simulink model "Assignment2_hardware_hiding"  (R2020a)
settings: Solver=FixedStepAuto  StartTime=0.0  StopTime=inf  FixedStep=1e-3  RelTol=1e-3  EnableMultiTasking=on
undefined symbols (not defined in the file or in its folder): A0, A1, D0, D1, D10, D11, D12, D13, D2, D3, D4, D5, D6, D7, D8, D9, PTA0, PTA1, PTA2, PTB2, PTB23, PTB3, PTB9, PTC16, PTC17, PTC2, PTC3, PTC4, PTD0, PTD1, PTD2, PTD3
libraries: frdmk64flib x22, etargetslib x7
settings Model: ExtModeTrigDuration=5  Creator=iceca  LastModifiedBy=iceca
settings OptimizationCC: EnhancedBackFolding=on  PassReuseOutputArgsAs=Individual arguments  ZeroExternalMemoryAtStartup=off  ZeroInternalMemoryAtStartup=off  MaxStackSize=64  OptimizeBlockOrder=speed  DifferentSizesBufferReuse=on  OptimizationCustomize=off  EfficientTunableParamExpr=on
settings DebuggingCC: ParameterTunabilityLossMsg=error
settings HardwareCC: ProdBitPerPointer=32  ProdBitPerSizeT=32  ProdBitPerPtrDiffT=32  ProdLargestAtomicInteger=Long  ProdLargestAtomicFloat=Double  ProdWordSize=32  ProdHWDeviceType=ARM Compatible->ARM Cortex
settings SFSimCC: MATLABDynamicMemAlloc=off
settings RTWCC: SystemTargetFile=ert.tlc  HardwareBoard=NXP FRDM-K64F  TemplateMakefile=ert_default_tmf  Toolchain=GNU Tools for ARM Embedded Processors
settings CodeAppCC: ForceParamTrailComments=on  IgnoreCustomStorageClasses=off  OperatorAnnotations=on  SimulinkDataObjDesc=on  SFDataObjDesc=on  InsertBlockDesc=on

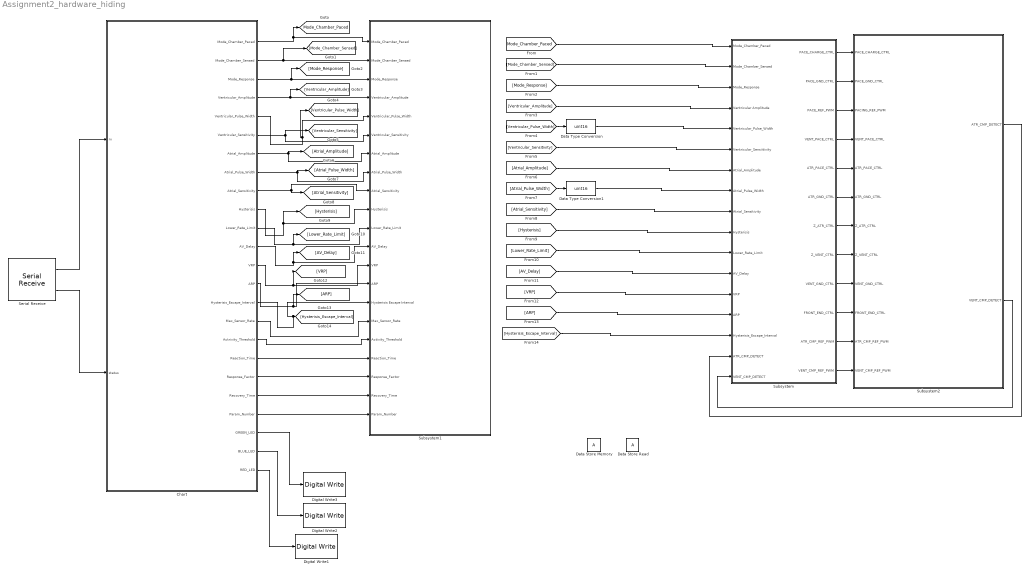
== system Assignment2_hardware_hiding ==
  Chart : Stateflow chart  TreatAsAtomicUnit=on
      settings: PortSchema="{\"entries\":[{\"content\":{\"sides\":[{\"content\":{\"connectorIds\":[\"In1\",\"In2\"]},\"type\":\"ConnectorPlacement.EquallySpacedRectSide\",\"uuid\":\"5d6148fe-63ad-4e41-a469-0ccea700ff5c\"},{\"content\":{\"connectorIds\":[\"Out1\",\"Out2\",\"Out3\",\"Out4\",\"Out5\",\"Out6\",\"Out7\",\"Out8\",\"Out9\",\"Out10\",\"Out11\",\"Out12\",\"Out13\",\"Out14\",\"Out15\",\"Out20\",\"Out21\",\"Out22\",\"Out23\",\"Out24\",\"Out18\",\"Out19\",\"Out16\",\"Out17\"],\"side\":\"RIGHT\"},\"type\":\"ConnectorPlacement.EquallySpacedRectSide\",\"uuid\":\"22e91669-c20d-44ca-9338-cd13d2e9e618\"},{\"content\":{\"connectorIds\":[],\"side\":\"TOP\"},\"type\":\"ConnectorPlacement.EquallySpacedRectSide\",\"uuid\":\"06f0f997-4aed-43a7-87af-d7ac7b59093d\"}]},\"type\":\"ConnectorPlacement.EquallySpacedConnector\",\"uuid\":\"618800eb-2d4f-49bb-a7f5-00e96badcb1e\"}],\"packageUris\":[\"http://schema.mathworks.com/mf0/Connector/19700101\"],\"version\":\"1.0\"}"
  Data Store Memory : DataStoreMemory  ReadBeforeWriteMsg=warning  WriteAfterWriteMsg=warning  WriteAfterReadMsg=warning  ShowAdditionalParam=off
  Data Store Read : DataStoreRead
  Data Type Conversion : DataTypeConversion  OutDataTypeStr=uint16
  Data Type Conversion1 : DataTypeConversion  OutDataTypeStr=uint16
  Digital Write1 : frdmk64flib/Digital Write  Whichpin=RED_LED
  Digital Write2 : frdmk64flib/Digital Write  Whichpin=BLUE_LED
  Digital Write3 : frdmk64flib/Digital Write  Whichpin=GREEN_LED
  Serial Receive : frdmk64flib/Serial Receive  SCIModule=0  Baudrate=uint32(9600)  Parity=None  StopBits=1  HardwareFlowControl=None  ByteOrder=LittleEndian  DataType=uint8  DataLength=27  BlockingMode=off  OutputStatus=on  SampleTime=-1
  Subsystem : Subsystem
  Subsystem1 : Subsystem
  Subsystem2 : Subsystem
  tag scope: Mode_Chamber_Paced=global
  wires:
  Serial Receive/1 -> Chart/1(rx)
  Serial Receive/2 -> Chart/2(status)
  Chart/1(Mode_Chamber_Paced) -> [Mode_Chamber_Paced], Subsystem1/1(Mode_Chamber_Paced)
  Chart/10(Hysterisis) -> Subsystem1/10(Hysterisis), [Hysterisis]
  Chart/11(Lower_Rate_Limit) -> Subsystem1/11(Lower_Rate_Limit), [Lower_Rate_Limit]
  Chart/12(AV_Delay) -> [AV_Delay], Subsystem1/12(AV_Delay)
  Chart/13(VRP) -> [VRP], Subsystem1/13(VRP)
  Chart/14(ARP) -> [ARP], Subsystem1/14(ARP)
  Chart/15(Hysterisis_Escape_Interval) -> [Hysterisis_Escape_Interval], Subsystem1/15(Hysterisis Escape Interval)
  Chart/2(Mode_Chamber_Sensed) -> Subsystem1/2(Mode_Chamber_Sensed), [Mode_Chamber_Sensed]
  Chart/3(Mode_Response) -> Subsystem1/3(Mode_Response), [Mode_Response]
  Chart/4(Ventricular_Amplitude) -> [Ventricular_Amplitude], Subsystem1/4(Ventricular_Amplitude)
  Chart/6(Ventricular_Sensitivity) -> [Ventricular_Sensitivity], Subsystem1/6(Ventricular_Sensitivity)
  Chart/7(Atrial_Amplitude) -> Subsystem1/7(Atrial_Amplitude), [Atrial_Amplitude]
  Chart/9(Atrial_Sensitivity) -> [Atrial_Sensitivity], Subsystem1/9(Atrial_Sensitivity)
  [Ventricular_Amplitude] -> Subsystem/4(Ventricular Amplitude)
  [Mode_Chamber_Sensed] -> Subsystem/2(Mode_Chamber_Sensed)
  [Mode_Chamber_Paced] -> Subsystem/1(Mode_Chamber_Paced)
  [Mode_Response] -> Subsystem/3(Mode_Response)
  [Ventricular_Sensitivity] -> Subsystem/6(Ventricular_Sensiitivity)
  [Atrial_Amplitude] -> Subsystem/7(Atrial_Amplitude)
  [Hysterisis] -> Subsystem/10(Hysterisis)
  [Lower_Rate_Limit] -> Subsystem/11(Lower_Rate_Limit)
  [AV_Delay] -> Subsystem/12(AV_Delay)
  [VRP] -> Subsystem/13(VRP)
  [ARP] -> Subsystem/14(ARP)
  [Hysterisis_Escape_Interval] -> Subsystem/15(Hysterisis_Escape_Interval)
  Chart/16(BLUE_LED) -> Digital Write2/1
  Chart/5(Ventricular_Pulse_Width) -> Subsystem1/5(Ventricular_Pulse_Width), [Ventricular_Pulse_Width]
  Chart/8(Atrial_Pulse_Width) -> [Atrial_Pulse_Width], Subsystem1/8(Atrial_Pulse_Width)
  [Ventricular_Pulse_Width] -> Data Type Conversion/1
  Data Type Conversion/1 -> Subsystem/5(Ventricular_Pulse_Width)
  [Atrial_Sensitivity] -> Subsystem/9(Atrial_Sensitivity)
  [Atrial_Pulse_Width] -> Data Type Conversion1/1
  Data Type Conversion1/1 -> Subsystem/8(Atrial_Pulse_Width)
  Chart/17(RED_LED) -> Digital Write1/1
  Chart/19(GREEN_LED) -> Digital Write3/1
  Chart/20(Max_Sensor_Rate) -> Subsystem1/16(Max_Sensor_Rate)
  Chart/21(Actrivity_Threshold) -> Subsystem1/17(Activity_Threshold)
  Chart/18(Param_Number) -> Subsystem1/21(Param_Number)
  Chart/24(Recovery_Time) -> Subsystem1/20(Recovery_Time)
  Chart/22(Reaction_Time) -> Subsystem1/18(Reaction_Time)
  Chart/23(Response_Factor) -> Subsystem1/19(Response_Factor)
  Subsystem2/2(VENT_CMP_DETECT) -> Subsystem/17(VENT_CMP_DETECT)
  Subsystem2/1(ATR_CMP_DETECT) -> Subsystem/16(ATR_CMP_DETECT)
  Subsystem/2(PACE_GND_CTRL) -> Subsystem2/2(PACE_GND_CTRL)
  Subsystem/4(VENT_PACE_CTRL) -> Subsystem2/4(VENT_PACE_CTRL)
  Subsystem/3(PACE_REF_PWM) -> Subsystem2/3(PACING_REF_PWM)
  Subsystem/1(PACE_CHARGE_CTRL) -> Subsystem2/1(PACE_CHARGE_CTRL)
  Subsystem/5(ATR_PACE_CTRL) -> Subsystem2/5(ATR_PACE_CTRL)
  Subsystem/6(ATR_GND_CTRL) -> Subsystem2/6(ATR_GND_CTRL)
  Subsystem/7(Z_ATR_CTRL) -> Subsystem2/7(Z_ATR_CTRL)
  Subsystem/8(Z_VENT_CTRL) -> Subsystem2/8(Z_VENT_CTRL)
  Subsystem/9(VENT_GND_CTRL) -> Subsystem2/9(VENT_GND_CTRL)
  Subsystem/10(FRONT_END_CTRL) -> Subsystem2/10(FRONT_END_CTRL)
  Subsystem/11(ATR_CMP_REF_PWM) -> Subsystem2/11(ATR_CMP_REF_PWM)
  Subsystem/12(VENT_CMP_REF_PWM) -> Subsystem2/12(VENT_CMP_REF_PWM)

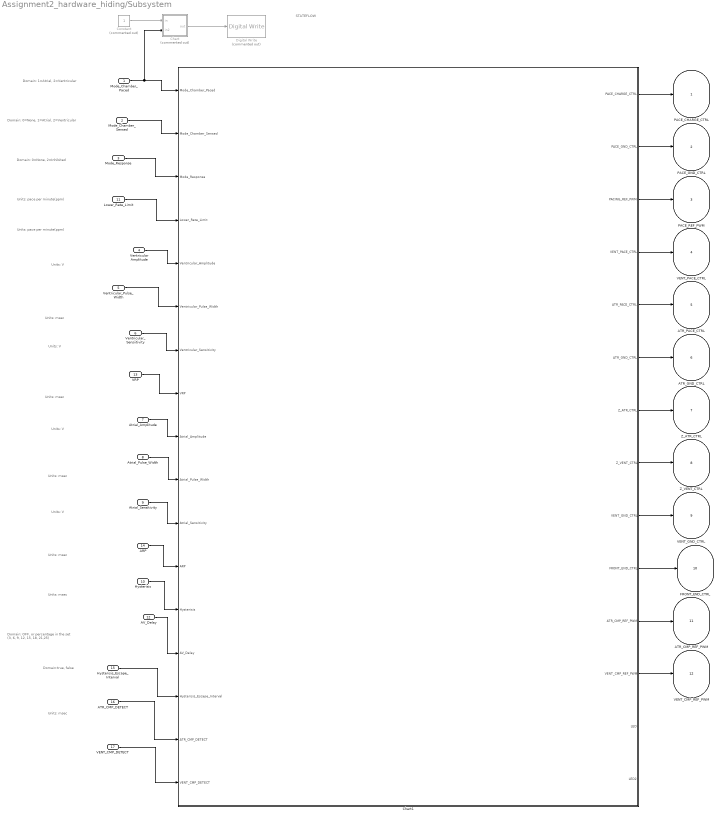
== system Assignment2_hardware_hiding/Subsystem ==
  note: Domain: OFF, or percentage
      | in the set (3, 6, 9, 12, 15, 18, 21,25)
  note: Domain: 0=None, 2=Inhibited
  note: Domain: 1=Atrial, 2=Ventricular
  note: Units: msec
  note: Units: pace per minute(ppm)
  note: Units: V
  note: STATEFLOW
  note: Units: msec
  note: Units: V
  note: Domain: 0=None, 1=Atrial, 2=Ventricular
  note: Units: pace per minute(ppm)
  note: Units: msec
  note: Units: msec
  note: Domain:true, false
  note: Units: V
  note: Units: msec
  note: Units: msec
  note: Units: V
  Mode_Chamber_Paced : Inport
  Mode_Chamber_Sensed : Inport  Port=2
  Mode_Response : Inport  Port=3
  Ventricular Amplitude : Inport  Port=4
  Ventricular_Pulse_Width : Inport  Port=5
  Ventricular_Sensiitivity : Inport  Port=6
  Atrial_Amplitude : Inport  Port=7
  Atrial_Pulse_Width : Inport  Port=8
  Atrial_Sensitivity : Inport  Port=9
  Hysterisis : Inport  Port=10
  Lower_Rate_Limit : Inport  Port=11
  AV_Delay : Inport  Port=12
  VRP : Inport  Port=13
  ARP : Inport  Port=14
  Hysterisis_Escape_Interval : Inport  Port=15
  ATR_CMP_DETECT : Inport  Port=16
  VENT_CMP_DETECT : Inport  Port=17
  Chart : Stateflow chart  Commented=on  TreatAsAtomicUnit=on
  Chart1 : Stateflow chart  TreatAsAtomicUnit=on
      settings: PortSchema="{\"entries\":[{\"content\":{\"sides\":[{\"content\":{\"connectorIds\":[\"In1\",\"In2\",\"In3\",\"In4\",\"In5\",\"In6\",\"In7\",\"In8\",\"In9\",\"In10\",\"In11\",\"In12\",\"In13\",\"In17\",\"In14\",\"In15\",\"In16\"]},\"type\":\"ConnectorPlacement.EquallySpacedRectSide\",\"uuid\":\"ef801456-a3d3-4c00-800f-18f55ff1f97a\"},{\"content\":{\"connectorIds\":[\"Out1\",\"Out2\",\"Out3\",\"Out4\",\"Out5\",\"Out6\",\"Out7\",\"Out8\",\"Out9\",\"Out10\",\"Out11\",\"Out12\",\"Out13\",\"Out14\"],\"side\":\"RIGHT\"},\"type\":\"ConnectorPlacement.EquallySpacedRectSide\",\"uuid\":\"5ac52b61-bf48-4a4b-86f3-012ecfccb962\"},{\"content\":{\"connectorIds\":[],\"side\":\"TOP\"},\"type\":\"ConnectorPlacement.EquallySpacedRectSide\",\"uuid\":\"b91e78a1-d42c-4358-92cf-ad767f596c0a\"}]},\"type\":\"ConnectorPlacement.EquallySpacedConnector\",\"uuid\":\"810cd47a-6ba0-4b6e-85f5-59d182ca7955\"}],\"packageUris\":[\"http://schema.mathworks.com/mf0/Connector/19700101\"],\"version\":\"1.0\"}"
  Constant : Constant  Commented=on
  Digital Write : frdmk64flib/Digital Write  Commented=on  Whichpin=RED_LED
  PACE_CHARGE_CTRL : Outport
  PACE_GND_CTRL : Outport  Port=2
  PACE_REF_PWM : Outport  Port=3
  VENT_PACE_CTRL : Outport  Port=4
  ATR_PACE_CTRL : Outport  Port=5
  ATR_GND_CTRL : Outport  Port=6
  Z_ATR_CTRL : Outport  Port=7
  Z_VENT_CTRL : Outport  Port=8
  VENT_GND_CTRL : Outport  Port=9
  FRONT_END_CTRL : Outport  Port=10
  ATR_CMP_REF_PWM : Outport  Port=11
  VENT_CMP_REF_PWM : Outport  Port=12
  wires:
  Hysterisis/1 -> Chart1/13(Hysterisis)
  Hysterisis_Escape_Interval/1 -> Chart1/14(Hysterisis_Escape_Interval)
  Ventricular_Pulse_Width/1 -> Chart1/6(Ventricular_Pulse_Width)
  Mode_Chamber_Paced/1 -> Chart1/1(Mode_Chamber_Paced), Chart/2(in2)
  Mode_Chamber_Sensed/1 -> Chart1/2(Mode_Chamber_Sensed)
  Mode_Response/1 -> Chart1/3(Mode_Response)
  ARP/1 -> Chart1/12(ARP)
  Lower_Rate_Limit/1 -> Chart1/4(Lower_Rate_Limit)
  Ventricular Amplitude/1 -> Chart1/5(Ventricular_Amplitude)
  Ventricular_Sensiitivity/1 -> Chart1/7(Ventricular_Sensitivity)
  VRP/1 -> Chart1/8(VRP)
  Atrial_Amplitude/1 -> Chart1/9(Atrial_Amplitude)
  Atrial_Pulse_Width/1 -> Chart1/10(Atrial_Pulse_Width)
  Atrial_Sensitivity/1 -> Chart1/11(Atrial_Sensitivity)
  Constant/1 -> Chart/1(in)
  Chart/1(out) -> Digital Write/1
  AV_Delay/1 -> Chart1/17(AV_Delay)
  ATR_CMP_DETECT/1 -> Chart1/15(ATR_CMP_DETECT)
  VENT_CMP_DETECT/1 -> Chart1/16(VENT_CMP_DETECT)
  Chart1/1(PACE_CHARGE_CTRL) -> PACE_CHARGE_CTRL/1
  Chart1/2(PACE_GND_CTRL) -> PACE_GND_CTRL/1
  Chart1/3(PACING_REF_PWM) -> PACE_REF_PWM/1
  Chart1/4(VENT_PACE_CTRL) -> VENT_PACE_CTRL/1
  Chart1/5(ATR_PACE_CTRL) -> ATR_PACE_CTRL/1
  Chart1/6(ATR_GND_CTRL) -> ATR_GND_CTRL/1
  Chart1/7(Z_ATR_CTRL) -> Z_ATR_CTRL/1
  Chart1/8(Z_VENT_CTRL) -> Z_VENT_CTRL/1
  Chart1/9(VENT_GND_CTRL) -> VENT_GND_CTRL/1
  Chart1/10(FRONT_END_CTRL) -> FRONT_END_CTRL/1
  Chart1/11(ATR_CMP_REF_PWM) -> ATR_CMP_REF_PWM/1
  Chart1/12(VENT_CMP_REF_PWM) -> VENT_CMP_REF_PWM/1

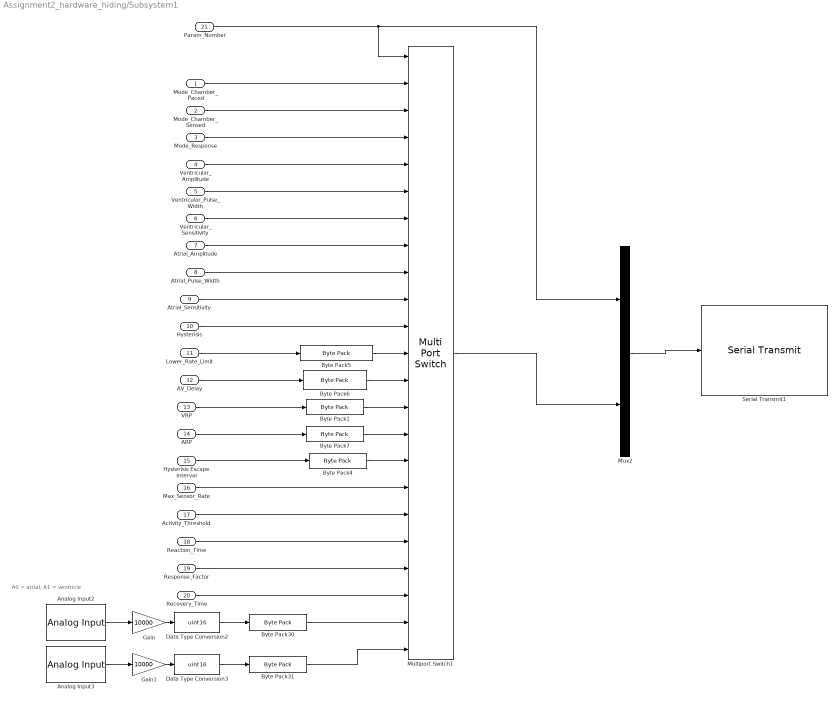
== system Assignment2_hardware_hiding/Subsystem1 ==
  note: A0 = atrial, A1 = ventricle
  Mode_Chamber_Paced : Inport
  Mode_Chamber_Sensed : Inport  Port=2
  Mode_Response : Inport  Port=3
  Ventricular_Amplitude : Inport  Port=4
  Ventricular_Pulse_Width : Inport  Port=5
  Ventricular_Sensitivity : Inport  Port=6
  Atrial_Amplitude : Inport  Port=7
  Atrial_Pulse_Width : Inport  Port=8
  Atrial_Sensitivity : Inport  Port=9
  Hysterisis : Inport  Port=10
  Lower_Rate_Limit : Inport  Port=11
  AV_Delay : Inport  Port=12
  VRP : Inport  Port=13
  ARP : Inport  Port=14
  Hysterisis Escape Interval : Inport  Port=15
  Max_Sensor_Rate : Inport  Port=16
  Activity_Threshold : Inport  Port=17
  Reaction_Time : Inport  Port=18
  Response_Factor : Inport  Port=19
  Recovery_Time : Inport  Port=20
  Param_Number : Inport  Port=21
  Analog Input2 : frdmk64flib/Analog Input  Whichpin=PTB2 (A0)  SampleTime=-1
  Analog Input3 : frdmk64flib/Analog Input  Whichpin=PTB3 (A1)  SampleTime=-1
  Byte Pack{1,4..7,30..31} (7 alike) : etargetslib/Byte Pack  datatypes={'uint16'}  byteAlign=1
  Data Type Conversion2 : DataTypeConversion  OutDataTypeStr=uint16
  Data Type Conversion3 : DataTypeConversion  OutDataTypeStr=uint16
  Gain : Gain  Gain=10000
  Gain1 : Gain  Gain=10000
  Multiport Switch1 : MultiPortSwitch  Inputs=22
  Mux2 : Mux  Inputs=2
  Serial Transmit1 : frdmk64flib/Serial Transmit  SCIModule=0  Baudrate=uint32(9600)  Parity=None  StopBits=1  HardwareFlowControl=None  ByteOrder=LittleEndian  BlockingMode=on  OutputStatus=off
  wires:
  Lower_Rate_Limit/1 -> Byte Pack5/1
  ARP/1 -> Byte Pack7/1
  VRP/1 -> Byte Pack1/1
  Hysterisis Escape Interval/1 -> Byte Pack4/1
  AV_Delay/1 -> Byte Pack6/1
  Param_Number/1 -> Mux2/1, Multiport Switch1/1
  Mode_Response/1 -> Multiport Switch1/4
  Mode_Chamber_Sensed/1 -> Multiport Switch1/3
  Mode_Chamber_Paced/1 -> Multiport Switch1/2
  Ventricular_Amplitude/1 -> Multiport Switch1/5
  Ventricular_Pulse_Width/1 -> Multiport Switch1/6
  Ventricular_Sensitivity/1 -> Multiport Switch1/7
  Atrial_Amplitude/1 -> Multiport Switch1/8
  Atrial_Pulse_Width/1 -> Multiport Switch1/9
  Atrial_Sensitivity/1 -> Multiport Switch1/10
  Hysterisis/1 -> Multiport Switch1/11
  Byte Pack5/1 -> Multiport Switch1/12
  Byte Pack6/1 -> Multiport Switch1/13
  Byte Pack1/1 -> Multiport Switch1/14
  Byte Pack7/1 -> Multiport Switch1/15
  Byte Pack4/1 -> Multiport Switch1/16
  Max_Sensor_Rate/1 -> Multiport Switch1/17
  Activity_Threshold/1 -> Multiport Switch1/18
  Reaction_Time/1 -> Multiport Switch1/19
  Response_Factor/1 -> Multiport Switch1/20
  Recovery_Time/1 -> Multiport Switch1/21
  Multiport Switch1/1 -> Mux2/2
  Mux2/1 -> Serial Transmit1/1
  Analog Input2/1 -> Gain/1
  Gain/1 -> Data Type Conversion2/1
  Data Type Conversion2/1 -> Byte Pack30/1
  Byte Pack30/1 -> Multiport Switch1/22
  Gain1/1 -> Data Type Conversion3/1
  Data Type Conversion3/1 -> Byte Pack31/1
  Analog Input3/1 -> Gain1/1
  Byte Pack31/1 -> Multiport Switch1/23

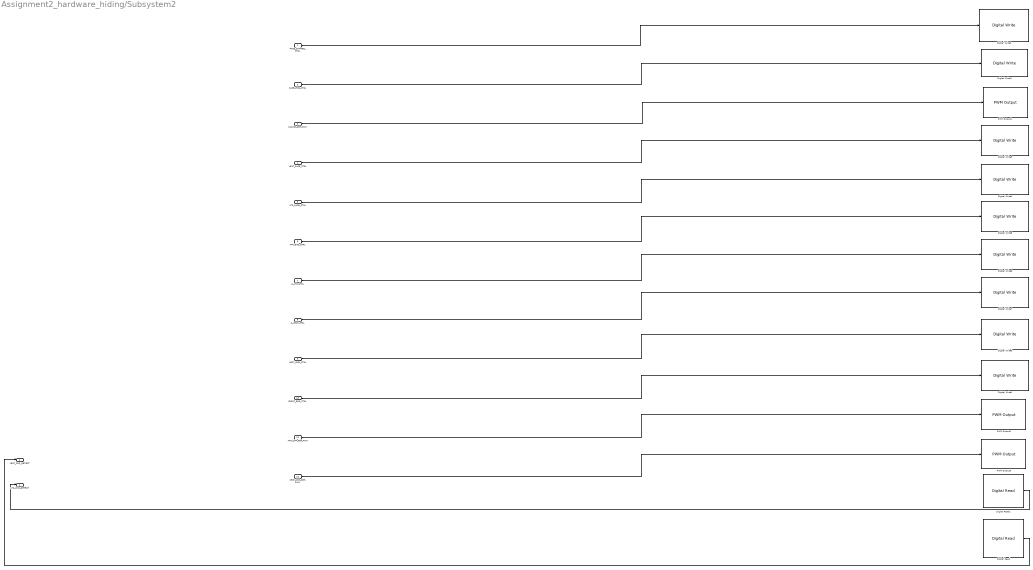
== system Assignment2_hardware_hiding/Subsystem2 ==
  PACE_CHARGE_CTRL : Inport
  PACE_GND_CTRL : Inport  Port=2
  PACING_REF_PWM : Inport  Port=3
  VENT_PACE_CTRL : Inport  Port=4
  ATR_PACE_CTRL : Inport  Port=5
  ATR_GND_CTRL : Inport  Port=6
  Z_ATR_CTRL : Inport  Port=7
  Z_VENT_CTRL : Inport  Port=8
  VENT_GND_CTRL : Inport  Port=9
  FRONT_END_CTRL : Inport  Port=10
  ATR_CMP_REF_PWM : Inport  Port=11
  VENT_CMP_REF_PWM : Inport  Port=12
  Digital Read : frdmk64flib/Digital Read  Whichpin=PTC16 (D0)  SampleTime=-1
  Digital Read1 : frdmk64flib/Digital Read  Whichpin=PTC17 (D1)  SampleTime=-1
  Digital Write1 : frdmk64flib/Digital Write  Whichpin=PTD1 (D13)
  Digital Write2 : frdmk64flib/Digital Write  Whichpin=PTB9 (D2)
  Digital Write3 : frdmk64flib/Digital Write  Whichpin=PTD0 (D10)
  Digital Write4 : frdmk64flib/Digital Write  Whichpin=PTA0 (D8)
  Digital Write5 : frdmk64flib/Digital Write  Whichpin=PTD2 (D11)
  Digital Write6 : frdmk64flib/Digital Write  Whichpin=PTB23 (D4)
  Digital Write7 : frdmk64flib/Digital Write  Whichpin=PTC3 (D7)
  Digital Write8 : frdmk64flib/Digital Write  Whichpin=PTC4 (D9)
  Digital Write9 : frdmk64flib/Digital Write  Whichpin=PTD3 (D12)
  PWM Output1 : frdmk64flib/PWM Output  Whichpin=PTA2 (D5)  InitialFrequency=2000  InitialDutyCycle=0
  PWM Output2 : frdmk64flib/PWM Output  Whichpin=PTC2 (D6)  InitialFrequency=2000  InitialDutyCycle=0
  PWM Output3 : frdmk64flib/PWM Output  Whichpin=PTA1 (D3)  InitialFrequency=2000  InitialDutyCycle=0
  ATR_CMP_DETECT : Outport
  VENT_CMP_DETECT : Outport  Port=2
  wires:
  PACING_REF_PWM/1 -> PWM Output1/1
  VENT_GND_CTRL/1 -> Digital Write9/1
  PACE_GND_CTRL/1 -> Digital Write3/1
  ATR_GND_CTRL/1 -> Digital Write5/1
  ATR_CMP_REF_PWM/1 -> PWM Output2/1
  VENT_PACE_CTRL/1 -> Digital Write8/1
  Digital Read1/1 -> ATR_CMP_DETECT/1
  Digital Read/1 -> VENT_CMP_DETECT/1
  VENT_CMP_REF_PWM/1 -> PWM Output3/1
  Z_VENT_CTRL/1 -> Digital Write7/1
  Z_ATR_CTRL/1 -> Digital Write6/1
  PACE_CHARGE_CTRL/1 -> Digital Write2/1
  ATR_PACE_CTRL/1 -> Digital Write4/1
  FRONT_END_CTRL/1 -> Digital Write1/1

== stateflow chart Assignment2_hardware_hiding/Subsystem/Chart1 ==
  state A_CHARGING_V_DISCHARGING1
    entry:
    %charge atrium
    ATR_PACE_CTRL=LOW;
    VENT_PACE_CTRL=LOW;
    PACING_REF_PWM=Atrial_Amplitude;
    PACE_CHARGE_CTRL=HIGH;
    %discharge ventricle
    PACE_GND_CTRL=HIGH;
    VENT_PACE_CTRL=LOW;
    Z_ATR_CTRL=LOW;
    Z_VENT_CTRL=LOW;
    ATR_PACE_CTRL=LOW;
    ATR_GND_CTRL=LOW;
    VENT_GND_CTRL=HIGH;
    Atrial_Escape_Interval =Lower_Rate_Limit-AV_Delay;
    LED2=false;
  state A_PACING1
    entry:
    PACE_CHARGE_CTRL = LOW;
    PACE_GND_CTRL = HIGH;
    VENT_PACE_CTRL = LOW;
    ATR_GND_CTRL =LOW;
    Z_ATR_CTRL = LOW;
    Z_VENT_CTRL = LOW;
    VENT_GND_CTRL = LOW;
    ATR_PACE_CTRL =HIGH;
  state V_CHARGING_A_DISCHARGING1
    entry:
    %Charging c22
    ATR_PACE_CTRL=LOW;
    VENT_PACE_CTRL=LOW;
    PACING_REF_PWM=Ventricular_Amplitude;
    PACE_CHARGE_CTRL=HIGH;
    %Discharging Atrium
    PACE_GND_CTRL=HIGH;
    VENT_PACE_CTRL=LOW;
    Z_ATR_CTRL=LOW;
    Z_VENT_CTRL=LOW;
    ATR_PACE_CTRL=LOW;
    ATR_GND_CTRL=HIGH;
    VENT_GND_CTRL=LOW;
  state V_PACING1
    entry:
    PACE_CHARGE_CTRL = LOW;
    PACE_GND_CTRL = HIGH;
    ATR_PACE_CTRL = LOW;
    ATR_GND_CTRL =LOW;
    Z_ATR_CTRL = LOW;
    Z_VENT_CTRL = LOW;
    VENT_GND_CTRL = LOW;
    VENT_PACE_CTRL =HIGH;
  state DECIDE_STATEFLOW
    entry:
    LED2=true;
    LED=false;
  state Charging_C23
    entry:
    ATR_PACE_CTRL   = LOW;
    VENT_PACE_CTRL = LOW;
    LED2=false;
  state Atrial_Charge
    entry:
    PACING_REF_PWM = Atrial_Amplitude;
  state Ventricular_Charge
    entry:
    PACING_REF_PWM = Ventricular_Amplitude;
  state Discharging_C21_and_Pace_Interval_Calculations
    entry:
    PACE_CHARGE_CTRL = HIGH;
    %Discharging C21
    PACE_GND_CTRL=HIGH;
    VENT_PACE_CTRL=LOW;
    Z_ATR_CTRL= LOW;
    Z_VENT_CTRL = LOW;
    ATR_PACE_CTRL = LOW;
    Pace_Interval = Lower_Rate_Limit;
    if Hysterisis == HIGH
    Pace_Interval = Pace_Interval + Hysterisis_Escape_Interval;
    end
  state Atrial_Discharge
    entry:
    ATR_GND_CTRL= HIGH;
    VENT_GND_CTRL= LOW;
    Pace_Interval =Pace_Interval-Atrial_Pulse_Width;
  state Ventricular_Discharge
    entry:
    ATR_GND_CTRL = LOW;
    VENT_GND_CTRL = HIGH;
    Pace_Interval =Pace_Interval -Ventricular_Pulse_Width;
  state Atrial_Sensing
    entry:
    FRONT_END_CTRL = HIGH;
    ATR_CMP_REF_PWM= Atrial_Sensitivity;
  state Ventricular_Sensing
    entry:
    FRONT_END_CTRL = HIGH;
    VENT_CMP_REF_PWM = Ventricular_Sensitivity;
  state No_Natural_Activity_Sensed
    entry:
    FRONT_END_CTRL = HIGH;
  state Pacing_Begin
    entry:
    PACE_CHARGE_CTRL = LOW;
    PACE_GND_CTRL = HIGH;
  state Ventricular_Pacing
    entry:
    ATR_PACE_CTRL = LOW;
  state Atrial_Pacing
    entry:
    VENT_PACE_CTRL = LOW;
  state Pacing
    entry:
    ATR_GND_CTRL =LOW;
    Z_ATR_CTRL = LOW;
    Z_VENT_CTRL = LOW;
    VENT_GND_CTRL = LOW;
  state Vent_Pacing_2
    entry:
    VENT_PACE_CTRL =HIGH;
  state Atrial_Pacing_2
    entry:
    ATR_PACE_CTRL =HIGH;
  A_CHARGING_V_DISCHARGING1 -> A_PACING1 : [after(Atrial_Escape_Interval-Atrial_Pulse_Width-Ventricular_Pulse_Width, msec)]
  A_PACING1 -> V_CHARGING_A_DISCHARGING1 : [after(Atrial_Pulse_Width,msec)]
  DECIDE_STATEFLOW -> A_CHARGING_V_DISCHARGING1 [order 1] : [Mode_Chamber_Paced==3]
  V_CHARGING_A_DISCHARGING1 -> V_PACING1 : [after(AV_Delay,msec)]
  V_PACING1 -> DECIDE_STATEFLOW : [after(Ventricular_Pulse_Width,msec)]
  (default) -> DECIDE_STATEFLOW
  Ventricular_Sensing -> DECIDE_STATEFLOW [order 2] : [Mode_Response==2 &&  VENT_CMP_DETECT==true && after(VRP, msec)]
  Atrial_Pacing_2 -> DECIDE_STATEFLOW : [after(Atrial_Pulse_Width,msec)]
  Vent_Pacing_2 -> DECIDE_STATEFLOW : [after(Ventricular_Pulse_Width,msec)]
  Atrial_Sensing -> DECIDE_STATEFLOW [order 2] : [Mode_Response==2 && after(ARP, msec) && ATR_CMP_DETECT==HIGH]
  DECIDE_STATEFLOW -> Charging_C23 [order 2] : [Mode_Chamber_Paced==2 || Mode_Chamber_Paced==1]
  Charging_C23 -> Atrial_Charge [order 2] : [Mode_Chamber_Paced==1]
  Charging_C23 -> Ventricular_Charge [order 1] : [Mode_Chamber_Paced==2]
  Atrial_Charge -> Discharging_C21_and_Pace_Interval_Calculations
  Ventricular_Charge -> Discharging_C21_and_Pace_Interval_Calculations
  Discharging_C21_and_Pace_Interval_Calculations -> Ventricular_Discharge [order 2] : [Mode_Chamber_Paced==2]
  Discharging_C21_and_Pace_Interval_Calculations -> Atrial_Discharge [order 1] : [Mode_Chamber_Paced==1]
  Atrial_Discharge -> Atrial_Sensing [order 2] : [Mode_Chamber_Sensed==1]
  Atrial_Discharge -> No_Natural_Activity_Sensed [order 1] : [Mode_Chamber_Sensed==0 && after(Pace_Interval, msec)]
  Ventricular_Discharge -> No_Natural_Activity_Sensed [order 2] : [Mode_Chamber_Sensed==0 && after(Pace_Interval, msec)]
  Ventricular_Discharge -> Ventricular_Sensing [order 1] : [Mode_Chamber_Sensed==2]
  Atrial_Sensing -> No_Natural_Activity_Sensed [order 1] : [after(Pace_Interval,msec)]
  Ventricular_Sensing -> No_Natural_Activity_Sensed [order 1] : [after(Pace_Interval,msec)]
  No_Natural_Activity_Sensed -> Pacing_Begin
  Pacing_Begin -> Ventricular_Pacing [order 1] : [Mode_Chamber_Paced==2]
  Pacing_Begin -> Atrial_Pacing [order 2] : [Mode_Chamber_Paced==1]
  Atrial_Pacing -> Pacing
  Ventricular_Pacing -> Pacing
  Pacing -> Atrial_Pacing_2 [order 2] : [Mode_Chamber_Paced==1]
  Pacing -> Vent_Pacing_2 [order 1] : [Mode_Chamber_Paced==2]
  data: Mode_Chamber_Paced input; Mode_Chamber_Sensed input; Mode_Response input; PACE_CHARGE_CTRL output; PACE_GND_CTRL output; PACING_REF_PWM output; VENT_PACE_CTRL output; ATR_PACE_CTRL output; ATR_GND_CTRL output; Z_ATR_CTRL output; Z_VENT_CTRL output; VENT_GND_CTRL output; Lower_Rate_Limit input; HIGH local boolean =true; LOW local boolean =false; Ventricular_Amplitude input; Ventricular_Pulse_Width input; Ventricular_Sensitivity input; VRP input; Atrial_Amplitude input; Atrial_Pulse_Width input; Atrial_Sensitivity input; ARP input; FRONT_END_CTRL output; ATR_CMP_REF_PWM output; VENT_CMP_REF_PWM output; Hysterisis input; Hysterisis_Escape_Interval input; ATR_CMP_DETECT input; VENT_CMP_DETECT input; Pace_Interval local; LED output; LED2 output; AV_Delay input; Atrial_Escape_Interval local

== stateflow chart Assignment2_hardware_hiding/Subsystem/Chart ==
  state INVESTIGATE
    entry:
    if in == in2
    out = true;
    end
    if in~= in2
    out = false;
    end
  (default) -> INVESTIGATE
  data: in input; out output; in2 input

== stateflow chart Assignment2_hardware_hiding/Chart ==
  state SET_PARAMS
    entry:
    offset=3;
    RED_LED = true;
    %MODE
    Mode_Chamber_Paced=rx(offset);
    offset=offset+uint8_bytes;
    Mode_Chamber_Sensed=rx(offset);
    offset=offset+uint8_bytes;
    Mode_Response=rx(offset);
    offset=offset+uint8_bytes;
    %VENTRICLULAR PACE PARAMS
    Ventricular_Amplitude=rx(offset);
    offset=offset+uint8_bytes;
    Ventricular_Pulse_Width=rx(offset);
    offset=offset+uint8_bytes;
    Ventricular_Sensitivity=rx(offset);
    offset=offset+uint8_bytes;
    %ATRIAL PACE PARAMS
    Atrial_Amplitude=rx(offset);
    offset=offset+uint8_bytes;
    Atrial_Pulse_Width=rx(offset);
    offset=offset+uint8_bytes;
    Atrial_Sensitivity=rx(offset);
    offset=offset+uint8_bytes;
    %HYSTERISIS
    Hysterisis=rx(offset);
    offset=offset+uint8_bytes;
    %uint16 PARAMETERS
    Lower_Rate_Limit=typecast(rx(offset:offset+1),'uint16');
    offset=offset+uint16_bytes;
    AV_Delay=typecast(rx(offset:offset+1),'uint16');
    offset=offset+uint16_bytes;
    VRP=typecast(rx(offset:offset+1),'uint16');
    offset=offset+uint16_bytes;
    ARP=typecast(rx(offset:offset+1),'uint16');
    offset=offset+uint16_bytes;
    Hysterisis_Escape_Interval=typecast(rx(offset:offset+1),'uint16');
    offset=offset+uint16_bytes;
    %RATE ADAPTIVITY
    Max_Sensor_Rate = rx(offset);
    offset=offset+uint8_bytes;
    Actrivity_Threshold = rx(offset);
    offset=offset+uint8_bytes;
    Reaction_Time=rx(offset);
    offset=offset+uint8_bytes;
    Response_Factor = rx(offset);
    offset=offset+uint8_bytes;
    Recovery_Time =  rx(offset);
    offset=offset+uint8_bytes;
  note: TEST_CODE: 10
      | SET_CODE: 20
      | ECHO_CODE: 30
  state START_STATE
    entry:
    uint16_bytes = 2;
    uint8_bytes = 1;
    single_bytes=4;
  state WAIT_STATE
    entry:
    RED_LED=false;
    BLUE_LED=false;
    GREEN_LED=false;
  state DEAD [commented out]
    entry:
    RED_LED=true;
    BLUE_LED=true;
    GREEN_LED=true;
  state READ_PARAMS
    entry:
    GREEN_LED=true;
    Param_Number=rx(3);
    exit:
  SET_PARAMS -> WAIT_STATE
  (junction 199) -> SET_PARAMS [order 1] : [rx(2)==20]
  (default) -> START_STATE
  (junction 132) -> WAIT_STATE [order 2]
  START_STATE -> WAIT_STATE
  WAIT_STATE -> (junction 132) : [status == 0]
  (junction 132) -> (junction 199) [order 1] : [rx(1)==10]
  (junction 199) -> READ_PARAMS [order 2] : [rx(2) == 30]
  READ_PARAMS -> WAIT_STATE
  data: Mode_Chamber_Paced output; Mode_Chamber_Sensed output; Mode_Response output; Ventricular_Amplitude output; Ventricular_Pulse_Width output; Ventricular_Sensitivity output; Atrial_Amplitude output; rx input uint8; offset local; Atrial_Pulse_Width output; Atrial_Sensitivity output; Hysterisis output; Lower_Rate_Limit output; AV_Delay output; VRP output; ARP output; Hysterisis_Escape_Interval output; status input uint8; uint16_bytes local; uint8_bytes local; BLUE_LED output; RED_LED output; single_bytes local; Param_Number output; GREEN_LED output; Max_Sensor_Rate output; Actrivity_Threshold output; Reaction_Time output; Response_Factor output; Recovery_Time output
